simulink model "D53_LKAS_JLU_20200909_1612"  (R2018b)
settings: Solver=ode3  StartTime=0.0  StopTime=10.0  FixedStep=0.01  RelTol=1e-3  EnableMultiTasking=on
model workspace (MAT data in the model file):
  MCOS : class17 (value not decoded)
  MCOS : class17 (value not decoded)
  MCOS : class17 (value not decoded)
  MCOS : class17 (value not decoded)
  MCOS : class17 (value not decoded)
  MCOS : class17 (value not decoded)
  MCOS : class17 (value not decoded)
  MCOS : class17 (value not decoded)
  MCOS : class17 (value not decoded)
  MCOS : class17 (value not decoded)
  MCOS : class17 (value not decoded)
  MCOS : class17 (value not decoded)
  MCOS : class17 (value not decoded)
  MCOS : class17 (value not decoded)
  MCOS : class17 (value not decoded)
  MCOS : class17 (value not decoded)
  MCOS : class17 (value not decoded)
  MCOS : class17 (value not decoded)
  MCOS : class17 (value not decoded)
  MCOS : class17 (value not decoded)
  MCOS : class17 (value not decoded)
  MCOS : class17 (value not decoded)
  MCOS : class17 (value not decoded)
  MCOS : class17 (value not decoded)
  MCOS : class17 (value not decoded)
  MCOS : class17 (value not decoded)
  MCOS : class17 (value not decoded)
  MCOS : class17 (value not decoded)
  MCOS : class17 (value not decoded)
  MCOS : class17 (value not decoded)
  MCOS : class17 (value not decoded)
  MCOS : class17 (value not decoded)
  MCOS : class17 (value not decoded)
  MCOS : class17 (value not decoded)
  MCOS : class17 (value not decoded)
  MCOS : class17 (value not decoded)
  MCOS : class17 (value not decoded)
  MCOS : class17 (value not decoded)
  MCOS : class17 (value not decoded)
  MCOS : class17 (value not decoded)
  MCOS : class17 (value not decoded)
  MCOS : class17 (value not decoded)
  MCOS : class17 (value not decoded)
  MCOS : class17 (value not decoded)
  MCOS : class17 (value not decoded)
  MCOS : class17 (value not decoded)
  MCOS : class17 (value not decoded)
  MCOS : class17 (value not decoded)
  MCOS : class17 (value not decoded)
  MCOS : class17 (value not decoded)
  MCOS : class17 (value not decoded)
  MCOS : class17 (value not decoded)
  MCOS : class17 (value not decoded)
  MCOS : class17 (value not decoded)
  MCOS : class17 (value not decoded)
  MCOS : class17 (value not decoded)
  MCOS : class17 (value not decoded)
  MCOS : class17 (value not decoded)
  MCOS : class17 (value not decoded)
  MCOS : class17 (value not decoded)
  MCOS : class17 (value not decoded)
  MCOS : class17 (value not decoded)
  MCOS : class17 (value not decoded)
  MCOS : class17 (value not decoded)
  MCOS : class17 (value not decoded)
  MCOS : class17 (value not decoded)
  MCOS : class17 (value not decoded)
  MCOS : class17 (value not decoded)
  MCOS : class17 (value not decoded)
  MCOS : class17 (value not decoded)
  MCOS : class17 (value not decoded)
  MCOS : class17 (value not decoded)
  MCOS : class17 (value not decoded)
  MCOS : class17 (value not decoded)
  MCOS : class17 (value not decoded)
  MCOS : class17 (value not decoded)
  MCOS : class17 (value not decoded)
  MCOS : class17 (value not decoded)
  MCOS : class17 (value not decoded)
  MCOS : class17 (value not decoded)
  MCOS : class17 (value not decoded)
  MCOS : class17 (value not decoded)
  MCOS : class17 (value not decoded)
  MCOS : class17 (value not decoded)
  MCOS : class17 (value not decoded)
  MCOS : class17 (value not decoded)
  MCOS : class17 (value not decoded)
  MCOS : class17 (value not decoded)
  MCOS : class17 (value not decoded)
undefined symbols (not defined in the file): LKA_CarWidth, LKA_SampleTime, LKA_StrRatio_C, LKA_Veh2CamL_C, LKA_Veh2CamW_C, LKA_WhlBaseL_C, LL_CompSWA_C, LL_CrvtPrvwT_C, LL_DesDvt_C, LL_DvtComp_C, LL_DvtPrvwT_C, LL_DvtSpdDet_vDvtSpdMin_C, LL_HdAgExT_C, LL_HdAgPrvwT_C, LL_LAccMax_C, LL_LAccRMax_C, LL_LDW_EarliestWarnLine_C, LL_LDW_LatestWarnLine_C, LL_LDWS_SUPPRESS_HEADING, LL_LFClb_TFC_DiffCtlBalance, LL_LFClb_TFC_DiffCtrlMaxSWA, LL_LFClb_TFC_DiffCtrlRatio, LL_LFClb_TFC_facmGainLutGain1_C, LL_LFClb_TFC_facmGainLutGain2_C, LL_LFClb_TFC_facmIntegRatio, LL_LFClb_TFC_facmKlat_C, LL_LFClb_TFC_FfCtlRatio_C, LL_LFClb_TFC_phiIntegCtlMaxSWA_C, LL_LFClb_TFC_tiKlatPrvwT_C, LL_LFClb_TFC_vGainLutVehSpdLwr_C, LL_LFClb_TFC_vGainLutVehSpdUpr_C, LL_LKA_EarliestWarnLine_C, LL_LKA_LatestWarnLine_C, LL_LKAExPrcs_ExitC0Dvt, LL_LKAExPrcs_ExitC0Swt, LL_LKAExPrcs_tiExitTime1, LL_LKAExPrcs_tiExitTime2, LL_LKAExPrcs_tiExitTime3, LL_LKAS_OUT_OF_CONTROL_LAT_VEL, LL_LKAS_OUT_OF_CONTROL_TTLC, LL_LKASWASyn_M0, LL_LKASWASyn_M1, LL_LKASWASyn_M2, LL_LKASWASyn_M3K, LL_LKASWASyn_SWAaddMax, LL_LKASWASyn_T2, LL_LKASWASyn_tiTrqSwaRtTime, LL_LKASWASyn_tiTrqSwaTime, LL_LKASWASyn_TrqMax, LL_LKASWASyn_TrqSwaAddSwt, LL_LKASWASyn_TrqSwaRateDiff, LL_LSpdCompT_C, LL_lStpLngth_C, LL_MAX_DELAY_EPSSTAR_TIME, LL_MAX_DRIVER_TORQUE_DISABLE, LL_MAX_DRIVER_TORQUE_ENABLE, LL_MAX_LANE_WIDTH_DISABLE, LL_MAX_LANE_WIDTH_ENABLE, LL_MAX_LAT_ACC_DISABLE, LL_MAX_LAT_ACC_ENABLE ... (+30)
libraries: simulink x134, canmsglib x50, dspstat3 x3, simulink_extras x1
(part 7 of 17)

== system D53_LKAS_JLU_20200909_1612/LL/LL Inputs Mapping/bsVehMovInfo ==
  bsVehMovInfoIn : Inport
  Bus Creator : BusCreator  Inputs=10
  Bus Selector2 : BusSelector  OutputSignals=ESC_LatAcc,ESC_LatAcc_Valid,ESC_YawRate,ESC_YawRate_Valid,ESC_UnYawRate,ESC_VehSpd,ESC_LonAcc,ESC_LonAcc_Valid,ESC_Brake_Press,ESC_VehSpd_Valid
  bsVehMovInfoOut : Outport
  wires:
  bsVehMovInfoIn/1 -> Bus Selector2/1
  Bus Selector2/1 -> Bus Creator/1  "<ESC_LatAcc>"
  Bus Selector2/2 -> Bus Creator/2  "<ESC_LatAcc_Valid>"
  Bus Selector2/3 -> Bus Creator/3  "<ESC_YawRate>"
  Bus Selector2/4 -> Bus Creator/4  "<ESC_YawRate_Valid>"
  Bus Selector2/5 -> Bus Creator/5  "<ESC_UnYawRate>"
  Bus Selector2/6 -> Bus Creator/6  "<ESC_VehSpd>"
  Bus Selector2/7 -> Bus Creator/7  "<ESC_LonAcc>"
  Bus Selector2/8 -> Bus Creator/8  "<ESC_LonAcc_Valid>"
  Bus Selector2/9 -> Bus Creator/9  "<ESC_Brake_Press>"
  Bus Selector2/10 -> Bus Creator/10  "<ESC_VehSpd_Valid>"
  Bus Creator/1 -> bsVehMovInfoOut/1

== system D53_LKAS_JLU_20200909_1612/LL/LLOn/LDW ==
  LDW_stLDWActvFlg : Inport
  LDW_bsInInfoSyn : Inport  Port=2
  LDW_bsLDWClb : Inport  Port=3
  states : EnablePort  StatesWhenEnabling=reset
      settings: AttributesFormatString=states = %<StatesWhenEnabling>
  Bus Selector : BusSelector  OutputSignals=bsLaneInfo.bsL0Info.L0_C1,bsLaneInfo.bsR0Info.R0_C1
  Bus Selector1 : BusSelector  OutputSignals=LL_LDWS_SUPPRESS_HEADING
  Heading Angle Detection (HdAgDet) : Subsystem  Description=|
      | Block Name: Heading Angle Detection
      | Ab.: HdAgDet
      | No.: 1.3.1.0
      | Rev: 0.0.1
      | Update Date: 19-3-26
  LDWWarnInfo : MATLAB Function  TreatAsAtomicUnit=on
  LDW_Flag : Outport  OutputWhenDisabled=reset  InitialOutput=0
  wires:
  LDWWarnInfo/1(LDWWarnInfo) -> LDW_Flag/1
  Heading Angle Detection (HdAgDet)/1(HdAgDet_stHdAgDetFlg) -> LDWWarnInfo/2(LDW_stHdAgDetFlg)
  Bus Selector1/1 -> Heading Angle Detection (HdAgDet)/4(HdAgDet_phiHdAgThres_C)  "<LL_LDWS_SUPPRESS_HEADING>"
  LDW_bsLDWClb/1 -> Bus Selector1/1
  Bus Selector/2 -> Heading Angle Detection (HdAgDet)/3(HdAgDet_phiHdAgRgt)  "<R0_C1>"
  Bus Selector/1 -> Heading Angle Detection (HdAgDet)/2(HdAgDet_phiHdAgLft)  "<L0_C1>"
  LDW_stLDWActvFlg/1 -> LDWWarnInfo/1(LDW_stLDWActvFlg), Heading Angle Detection (HdAgDet)/1(HdAgDet_stLDWActvFlg)
  LDW_bsInInfoSyn/1 -> Bus Selector/1

== system D53_LKAS_JLU_20200909_1612/LL/LLOn/LKA ==
  LKA_bsInInfoSyn : Inport
  LKA_bsLKAInPInfo : Inport  Port=2
  LKA_bsLKAClb : Inport  Port=3
  LKA_bsConstantClb : Inport  Port=4
  states = reset : EnablePort  StatesWhenEnabling=reset  ShowOutputPort=on
  Bus Selector : BusSelector  OutputSignals=LKA_SampleTime
  Cast To Single : DataTypeConversion  OutDataTypeStr=uint8
  Driver Torque Addition (DTA) : Subsystem
  LKA Exit Processing (LKAExPrcs) : Subsystem  Description=|
      | Block Name: LKA Exit Processing 
      | Ab.: LKAExPrcs
      | No.: 1.2.2.0
      | Rev: 0.0.1
      | Update Date: 19-5-13
  "LKA Motion Planning (LKAMP) " : Subsystem  Description=|
      | Block Name: LKA Motion Planning
      | Ab.: LKAMP
      | No.: 1.2.3.0
      | Rev: 0.0.1
      | Update Date: 19-5-13
  LKA SWA Limit (LKASWALim) : Subsystem  Description=|
      | Block Name: LKA SWA Synthesis
      | Ab.: LKASWASyn
      | No.: 1.2.6.0
      | Rev: 0.0.1
      | Update Date: 19-5-13
  LKA_Mon : Subsystem
  Lane Following (LF) : Subsystem  Description=|
      | Block Name: Lane Following
      | Ab.: LF
      | No.: 02
      | Rev: 00.00.01
      | Update Date: 19-3-28
  Plan To LaneFollowing (PTLF) : Subsystem
  LKA_ExitFlg : Outport  OutputWhenDisabled=reset  InitialOutput=0
  LKA_phiSWACmd : Outport  Port=2  OutputWhenDisabled=reset  InitialOutput=0
  LKA_M : Outport  Port=3  OutputWhenDisabled=reset  InitialOutput=0
  LKAMon : Outport  Port=4  OutputWhenDisabled=reset  InitialOutput=0
  tag scope: ActFlg=global, Ff=global, LKA_ConstantClb=global, LKA_ExitFlg_Mon=global, LKA_SampleTime=global, PT1=global
  wires:
  LKA_Mon/1(LKAMon) -> LKAMon/1
  "LKA Motion Planning (LKAMP) "/2(LKAMP_tiT1) -> [PT1]  "PlanT1"
  "LKA Motion Planning (LKAMP) "/3(LKAMP_tiT2) -> ?  "PlanT2"
  "LKA Motion Planning (LKAMP) "/1(LKAMP_phiSWACmd) -> [Plan]  "PlanSWACmd"
  Lane Following (LF)/4(LF_phiDiffSWACmd) -> [D]
  Lane Following (LF)/2(LF_phiPropSWACmd) -> [P]
  Lane Following (LF)/1(LF_phiFfLFSWACmd) -> [Ff]
  Lane Following (LF)/3(LF_phiIntegSWACmd) -> [I]
  Driver Torque Addition (DTA)/2(DTA_M) -> LKA_M/1
  [LKAInPInfo] -> Lane Following (LF)/2(LF_bsLKAInPInfo)
  [Ff] -> LKA SWA Limit (LKASWALim)/2(LKASWALim_Ff)
  [LKA_bsInInfoSyn] -> Lane Following (LF)/1(LF_bsInInfoSyn)
  [LKA_bsInInfoSyn] -> Driver Torque Addition (DTA)/1(DTA_bsInInfoSyn)
  [LKA_bsInInfoSyn] -> "LKA Motion Planning (LKAMP) "/1(LKAMP_bsInInfoSyn)
  [LKA_bsInInfoSyn] -> LKA Exit Processing (LKAExPrcs)/1(LKAExPrcs_bsInInfoSyn)
  LKA_bsInInfoSyn/1 -> [LKA_bsInInfoSyn]
  [LKA_bsLKAClb] -> LKA SWA Limit (LKASWALim)/4(LKASWALim_bsLKAClb)
  [LKA_bsLKAClb] -> Lane Following (LF)/3(LF_bsLFClb)
  [LKA_bsLKAClb] -> Driver Torque Addition (DTA)/2(DTA_bsLFClb)
  [LKA_bsLKAClb] -> "LKA Motion Planning (LKAMP) "/4(LKAMP_bsLKAClb)
  [LKA_bsLKAClb] -> LKA Exit Processing (LKAExPrcs)/3(LKAExPrcs_bsLKAClb)
  [LKAInPInfo] -> LKA SWA Limit (LKASWALim)/3(LKASWALim_bsLKAInPInfo)
  LKA_bsLKAClb/1 -> [LKA_bsLKAClb]
  [LKAInPInfo] -> Plan To LaneFollowing (PTLF)/1(InP)
  [LKAInPInfo] -> LKA Exit Processing (LKAExPrcs)/2(LKAExPrcs_bsLKAInPInfo)
  [LKAInPInfo] -> "LKA Motion Planning (LKAMP) "/3(LKAMP_bsLKAInPInfo)
  LKA_bsLKAInPInfo/1 -> [LKAInPInfo]
  [LKA_ConstantClb] -> Lane Following (LF)/4(LF_bsConstantClb)
  [LKA_ConstantClb] -> "LKA Motion Planning (LKAMP) "/5(LLClb_bsConstantClb)
  [ActFlg] -> "LKA Motion Planning (LKAMP) "/2(LKAMP_stLKAActvFlg)
  [PT1] -> LKA Exit Processing (LKAExPrcs)/4(LKAExPrcs_PlanT1)
  [PT1] -> Plan To LaneFollowing (PTLF)/3(T1)
  [Plan] -> Plan To LaneFollowing (PTLF)/2(Plan)
  [DT] -> Plan To LaneFollowing (PTLF)/4(DrvTrq)
  Driver Torque Addition (DTA)/1(DTA_phiDTASWACmd) -> [DT]  "DT"
  [D] -> Plan To LaneFollowing (PTLF)/8(D)
  [I] -> Plan To LaneFollowing (PTLF)/7(I)
  [P] -> Plan To LaneFollowing (PTLF)/6(P)
  [Ff] -> Plan To LaneFollowing (PTLF)/5(Ff)
  LKA Exit Processing (LKAExPrcs)/1(LKAExPrcs_stExFlg) -> LKA_ExitFlg/1, [LKA_ExitFlg_Mon]
  LKA SWA Limit (LKASWALim)/1(LKASWALim_phiSWACmd) -> LKA_phiSWACmd/1  "phiSWACmd"
  states = reset/1 -> Cast To Single/1
  Plan To LaneFollowing (PTLF)/1(SWACmd) -> LKA SWA Limit (LKASWALim)/1(LKASWALim_phiTFCSWACmd)  "PTLFSWACmd"
  Cast To Single/1 -> [ActFlg]  "ActFlg"
  LKA_bsConstantClb/1 -> [LKA_ConstantClb], Bus Selector/1
  Bus Selector/1 -> [LKA_SampleTime]  "<LKA_SampleTime>"

== system D53_LKAS_JLU_20200909_1612/LL/LLOn/LKA Input Processing (LKAInP) ==
  LKAInP_stLKAActvFlg : Inport
  LKAInP_bsInInfoSyn : Inport  Port=2
  LKAInP_bsLKAClb : Inport  Port=3
  Bus Creator : BusCreator  Inputs=6
  Bus Creator1 : BusCreator  Inputs=3
  Delay : Delay  DelayLength=1
  Lane Width Calculation (LW) : Subsystem
  Predicted Deviation Calculation (PrDvt) : Subsystem
  Predicted Heading Angle Calculation (PrHdAg) : Subsystem
  Previewed Curvature (PrCrvt) : Subsystem
  Steering Wheel Position Calculation (SWAPosCal) : Subsystem
  TTLC Calculation (TTLCCalc) : Subsystem  Description=|
      | Block Name: TTLC Calculation
      | Ab.: TTLCCalc
      | No.: 1.1.1.1
      | Rev: 0.0.1
      | Update Date: 19-3-26
  Under The Limit (UndrLim) : Subsystem
  LKAInP_bsLKAInPInfo : Outport
  wires:
  TTLC Calculation (TTLCCalc)/1(TTLCCalc_bsTTLCInfo) -> Predicted Heading Angle Calculation (PrHdAg)/1(PrHdAg_bsTTLCInfo), Bus Creator/2  "TTLC_bsTTLCInfo"
  Lane Width Calculation (LW)/1(LW_LaneWidth) -> Bus Creator/1  "LW_LaneWidth"
  Steering Wheel Position Calculation (SWAPosCal)/1(SWAPosCal) -> Bus Creator/6  "LKAInP_phiSWAPos"
  LKAInP_stLKAActvFlg/1 -> Delay/1
  Under The Limit (UndrLim)/2(UndrLim_dphiSWARMax) -> Bus Creator/5  "UndrLim_dphiSWARMax"
  Under The Limit (UndrLim)/1(UndrLim_phiSWAMax) -> Bus Creator/4  "UndrLim_phiSWAMax"
  Bus Creator1/1 -> Bus Creator/3  "Pr_bsPrInfo"
  Previewed Curvature (PrCrvt)/1(PrvwCrvt_bsPrvwCrvtInfo) -> Bus Creator1/3, TTLC Calculation (TTLCCalc)/3(bsPrvwCrvtInfo)  "bsPrCrvtInfo"
  Predicted Deviation Calculation (PrDvt)/1(PrdcDvt_bsPrdcDvtInfo) -> Bus Creator1/1, TTLC Calculation (TTLCCalc)/2(bsPrDvtInfo)  "bsPrDvtInfo"
  Predicted Heading Angle Calculation (PrHdAg)/1(PrHdAg_bsPrHdAgInfo) -> Bus Creator1/2, Predicted Deviation Calculation (PrDvt)/3(PrdcDvt_bsPrdcHdAgInfo)  "bsPrHdAgInfo"
  LKAInP_bsLKAClb/1 -> Predicted Deviation Calculation (PrDvt)/4(PrdcDvt_bsLKAClb), Predicted Heading Angle Calculation (PrHdAg)/4(PrHdAg_bsLKAClb), Previewed Curvature (PrCrvt)/3(PrvwCrvt_tiCrvtPrvwT_C), Under The Limit (UndrLim)/2(UndrLim_bsUndrLimClb)
  Bus Creator/1 -> LKAInP_bsLKAInPInfo/1
  LKAInP_bsInInfoSyn/1 -> Lane Width Calculation (LW)/1(LW_bsInInfoSyn), TTLC Calculation (TTLCCalc)/1(bsInfo), Predicted Deviation Calculation (PrDvt)/2(PrdcDvt_bsInInfoSyn), Predicted Heading Angle Calculation (PrHdAg)/3(PrHdAg_bsInInfoSyn), Previewed Curvature (PrCrvt)/2(PrvwCrvt_bsInInfoSyn), Under The Limit (UndrLim)/1(UndrLim_bsInInfoSyn), Steering Wheel Position Calculation (SWAPosCal)/1(SWAPosCal_bsInInfoSyn)
  Delay/1 -> Predicted Deviation Calculation (PrDvt)/1(PrdcDvt_stLKAActvFlg), Predicted Heading Angle Calculation (PrHdAg)/2(PrdcHdAg_stLKAActvFlg), Previewed Curvature (PrCrvt)/1(PrvwCrvt_stLKAActvFlg)

== system D53_LKAS_JLU_20200909_1612/LL/LLOn/LL State Determination (LLStateDet) ==
  LLStateDet_stDACMode : Inport
  LLStateDet_bsInInfoSyn : Inport  Port=2
  LLStateDet_bsLKAInPInfo : Inport  Port=3
  LLStateDet_bsLLSMConClb : Inport  Port=4
  LLStateDet_stExitFlg : Inport  Port=5
  LLStateDet_SignalFault : Inport  Port=6
  Bus Creator : BusCreator  Inputs=3
  Delay : Delay  DelayLength=1
  Delay1 : Delay  DelayLength=1
  LDW_State_Machine : Stateflow chart  Description=|  TreatAsAtomicUnit=on
      | Block Name: LDW State Machine
      | Ab.: LDWSM
      | No.: 1.1.2.0
      | Rev: 0.0.1
      | Update Date: 19-3-26
      settings: RTWSystemCode=Nonreusable function
  LKA_State_Machine : Stateflow chart  Description=|  TreatAsAtomicUnit=on
      | Block Name: LKA State Machine
      | Ab.: LKASM
      | No.: 1.1.3.0
      | Rev: 0.0.1
      | Update Date: 19-3-26
      settings: RTWSystemCode=Nonreusable function
  LL State Machine Conditions (LLSMCon) : Subsystem
  LLStateDet_bsLLState : Outport
  LLStateDet_stLDWActvFlg : Outport  Port=2
  LLStateDet_stLKAActvFlg : Outport  Port=3
  tag scope: LDW_State_Mon=global, LKA_State_Mon=global
  wires:
  LLStateDet_SignalFault/1 -> LL State Machine Conditions (LLSMCon)/7(LLSMCon_bsSignalFault)
  Delay/1 -> LL State Machine Conditions (LLSMCon)/6(LLSMCon_stExitFlg)
  LLStateDet_bsLLSMConClb/1 -> LL State Machine Conditions (LLSMCon)/4(LLSMCon_bsLLSMConClb)
  LLStateDet_stExitFlg/1 -> Delay/1
  LLStateDet_stDACMode/1 -> LL State Machine Conditions (LLSMCon)/1(LLSMCon_stDACModeIn)
  LLStateDet_bsLKAInPInfo/1 -> LL State Machine Conditions (LLSMCon)/3(LLSMCon_bsLKAInPInfo)
  LLStateDet_bsInInfoSyn/1 -> LL State Machine Conditions (LLSMCon)/2(LLSMCon_bsInInfoSyn)
  LL State Machine Conditions (LLSMCon)/11(LLSMCon_stLKAFaultCSyn) -> LKA_State_Machine/6(LKASM_stFaultCSyn)
  LL State Machine Conditions (LLSMCon)/10(LLSMCon_stLKADeactvCSyn) -> LKA_State_Machine/5(LKASM_stDeactvCSyn)
  LL State Machine Conditions (LLSMCon)/9(LLSMCon_stLKAActvCSyn) -> LKA_State_Machine/4(LKASM_stActvCSyn)
  LL State Machine Conditions (LLSMCon)/8(LLSMCon_stLKADisblCSyn) -> LKA_State_Machine/3(LKASM_stDisblCSyn)
  LL State Machine Conditions (LLSMCon)/7(LLSMCon_stLKAEnaCSyn) -> LKA_State_Machine/2(LKASM_stEnaCSyn)
  LL State Machine Conditions (LLSMCon)/6(LLSMCon_stLDWFaultCSyn) -> LDW_State_Machine/6(LDWSM_stFaultCSyn)
  LDW_State_Machine/2(LDWSM_stLDWState) -> Bus Creator/1, [LDW_State_Mon]  "LDW_State"
  LKA_State_Machine/2(LKASM_stLKAState) -> Bus Creator/3, [LKA_State_Mon]  "LKA_State"
  Bus Creator/1 -> LLStateDet_bsLLState/1, Delay1/1  "LLState"
  Delay1/1 -> LL State Machine Conditions (LLSMCon)/5(LLSMCon_bsLLState)
  LKA_State_Machine/1(LKASM_stLKAActvFlg) -> LLStateDet_stLKAActvFlg/1
  LDW_State_Machine/1(LDWSM_stLDWActvFlg) -> LLStateDet_stLDWActvFlg/1
  LL State Machine Conditions (LLSMCon)/1(LLSMCon_stDACMode) -> LDW_State_Machine/1(LDWSM_stLMCMode), Bus Creator/2, LKA_State_Machine/1(LKASM_stLMCMode)  "DACMode"
  LL State Machine Conditions (LLSMCon)/5(LLSMCon_stLDWDeactvCSyn) -> LDW_State_Machine/5(LDWSM_stDeactvCSyn)
  LL State Machine Conditions (LLSMCon)/4(LLSMCon_stLDWActvCSyn) -> LDW_State_Machine/4(LDWSM_stActvCSyn)
  LL State Machine Conditions (LLSMCon)/3(LLSMCon_stLDWDisblCSyn) -> LDW_State_Machine/3(LDWSM_stDisblCSyn)
  LL State Machine Conditions (LLSMCon)/2(LLSMCon_stLDWEnaCSyn) -> LDW_State_Machine/2(LDWSM_stEnaCSyn)

== system D53_LKAS_JLU_20200909_1612/LL/LLOn/LL_Mon ==
  LKAMon : Inport
  Bus : BusCreator  Inputs=3
  BusInP : BusCreator  Inputs=2
  BusState : BusCreator  Inputs=2
  LLMon : Outport
  wires:
  BusState/1 -> [StateMon]  "StateMon"
  BusInP/1 -> [InPMon]  "InPMon"
  [LKA_State_Mon] -> BusState/2  "LKA_State_Mon"
  [LDW_State_Mon] -> BusState/1  "LDW_State_Mon"
  [RGTTTLC_Mon] -> BusInP/2  "RGTTTLC_Mon"
  [LFTTTLC_Mon] -> BusInP/1  "LFTTTLC_Mon"
  Bus/1 -> LLMon/1  "LLMon"
  LKAMon/1 -> Bus/3
  [StateMon] -> Bus/2
  [InPMon] -> Bus/1

== system D53_LKAS_JLU_20200909_1612/LLClb/LLSMConClb/ICv to v ==
  In1 : Inport
  Add : Sum  Inputs=+-
  Constant : Constant  Value=2.5  OutDataTypeStr=single
  Gain : Gain  Gain=1/1.02
  Out1 : Outport
  wires:
  Gain/1 -> Out1/1
  Constant/1 -> Add/2
  Add/1 -> Gain/1
  In1/1 -> Add/1

== system D53_LKAS_JLU_20200909_1612/LLClb/LLSMConClb/ICv to v1 ==
  In1 : Inport
  Add : Sum  Inputs=+-
  Constant : Constant  Value=2.5  OutDataTypeStr=single
  Gain : Gain  Gain=1/1.02
  Out1 : Outport
  wires:
  In1/1 -> Add/1
  Add/1 -> Gain/1
  Constant/1 -> Add/2
  Gain/1 -> Out1/1

== system D53_LKAS_JLU_20200909_1612/LLClb/LLSMConClb/ICv to v2 ==
  In1 : Inport
  Add : Sum  Inputs=+-
  Constant : Constant  Value=2.5  OutDataTypeStr=single
  Gain : Gain  Gain=1/1.02
  Out1 : Outport
  wires:
  Gain/1 -> Out1/1
  Constant/1 -> Add/2
  Add/1 -> Gain/1
  In1/1 -> Add/1

== system D53_LKAS_JLU_20200909_1612/LLClb/LLSMConClb/ICv to v3 ==
  In1 : Inport
  Add : Sum  Inputs=+-
  Constant : Constant  Value=2.5  OutDataTypeStr=single
  Gain : Gain  Gain=1/1.02
  Out1 : Outport
  wires:
  In1/1 -> Add/1
  Add/1 -> Gain/1
  Constant/1 -> Add/2
  Gain/1 -> Out1/1

== system D53_LKAS_JLU_20200909_1612/LLClb/LLSMConClb/ICv to v4 ==
  In1 : Inport
  Add : Sum  Inputs=+-
  Constant : Constant  Value=2.5  OutDataTypeStr=single
  Gain : Gain  Gain=1/1.02
  Out1 : Outport
  wires:
  Gain/1 -> Out1/1
  Constant/1 -> Add/2
  Add/1 -> Gain/1
  In1/1 -> Add/1

== system D53_LKAS_JLU_20200909_1612/LLClb/LLSMConClb/ICv to v5 ==
  In1 : Inport
  Add : Sum  Inputs=+-
  Constant : Constant  Value=2.5  OutDataTypeStr=single
  Gain : Gain  Gain=1/1.02
  Out1 : Outport
  wires:
  In1/1 -> Add/1
  Add/1 -> Gain/1
  Constant/1 -> Add/2
  Gain/1 -> Out1/1

== system D53_LKAS_JLU_20200909_1612/Clb/Calibration1/Subsystem2/If Action Subsystem ==
  In1 : Inport
  Action Port : ActionPort  ActionType=then
  Out1 : Outport
  wires:
  In1/1 -> Out1/1

== system D53_LKAS_JLU_20200909_1612/Clb/Calibration1/Subsystem2/If Action Subsystem1 ==
  In1 : Inport
  Action Port : ActionPort  ActionType=elseif
  Out1 : Outport
  wires:
  In1/1 -> Out1/1

== system D53_LKAS_JLU_20200909_1612/Clb/Calibration1/Subsystem2/If Action Subsystem2 ==
  In1 : Inport
  Action Port : ActionPort  ActionType=elseif
  Out1 : Outport
  wires:
  In1/1 -> Out1/1

== system D53_LKAS_JLU_20200909_1612/Clb/Calibration1/Subsystem2/If Action Subsystem3 ==
  In1 : Inport
  Action Port : ActionPort  ActionType=elseif
  Out1 : Outport
  wires:
  In1/1 -> Out1/1

== system D53_LKAS_JLU_20200909_1612/Clb/Calibration1/Subsystem2/If Action Subsystem4 ==
  In1 : Inport
  Action Port : ActionPort  ActionType=elseif
  Out1 : Outport
  wires:
  In1/1 -> Out1/1

== system D53_LKAS_JLU_20200909_1612/Clb/Calibration1/Subsystem2/If Action Subsystem5 ==
  In1 : Inport
  Action Port : ActionPort  ActionType=elseif
  Out1 : Outport
  wires:
  In1/1 -> Out1/1

== system D53_LKAS_JLU_20200909_1612/Clb/Calibration1/Subsystem2/If Action Subsystem6 ==
  In1 : Inport
  Action Port : ActionPort  ActionType=elseif
  Out1 : Outport
  wires:
  In1/1 -> Out1/1

== system D53_LKAS_JLU_20200909_1612/Clb/Calibration1/Subsystem2/If Action Subsystem7 ==
  In1 : Inport
  Action Port : ActionPort  ActionType=elseif
  Out1 : Outport
  wires:
  In1/1 -> Out1/1

== system D53_LKAS_JLU_20200909_1612/Clb/Calibration1/Subsystem2/If Action Subsystem8 ==
  In1 : Inport
  Action Port : ActionPort  ActionType=elseif
  Out1 : Outport
  wires:
  In1/1 -> Out1/1

== system D53_LKAS_JLU_20200909_1612/Clb/Calibration1/Subsystem2/If Action Subsystem9 ==
  In1 : Inport
  Action Port : ActionPort  ActionType=elseif
  Out1 : Outport
  wires:
  In1/1 -> Out1/1

== system D53_LKAS_JLU_20200909_1612/Clb/Calibration2/Subsystem2/If Action Subsystem ==
  In1 : Inport
  Action Port : ActionPort  ActionType=then
  Out1 : Outport
  wires:
  In1/1 -> Out1/1

== system D53_LKAS_JLU_20200909_1612/Clb/Calibration2/Subsystem2/If Action Subsystem1 ==
  In1 : Inport
  Action Port : ActionPort  ActionType=elseif
  Out1 : Outport
  wires:
  In1/1 -> Out1/1

== system D53_LKAS_JLU_20200909_1612/Clb/Calibration2/Subsystem2/If Action Subsystem2 ==
  In1 : Inport
  Action Port : ActionPort  ActionType=elseif
  Out1 : Outport
  wires:
  In1/1 -> Out1/1

== system D53_LKAS_JLU_20200909_1612/Clb/Calibration2/Subsystem2/If Action Subsystem3 ==
  In1 : Inport
  Action Port : ActionPort  ActionType=elseif
  Out1 : Outport
  wires:
  In1/1 -> Out1/1

== system D53_LKAS_JLU_20200909_1612/Clb/Calibration2/Subsystem2/If Action Subsystem4 ==
  In1 : Inport
  Action Port : ActionPort  ActionType=elseif
  Out1 : Outport
  wires:
  In1/1 -> Out1/1

== system D53_LKAS_JLU_20200909_1612/Clb/Calibration2/Subsystem2/If Action Subsystem5 ==
  In1 : Inport
  Action Port : ActionPort  ActionType=elseif
  Out1 : Outport
  wires:
  In1/1 -> Out1/1

== system D53_LKAS_JLU_20200909_1612/Clb/Calibration2/Subsystem2/If Action Subsystem6 ==
  In1 : Inport
  Action Port : ActionPort  ActionType=elseif
  Out1 : Outport
  wires:
  In1/1 -> Out1/1

== system D53_LKAS_JLU_20200909_1612/Clb/Calibration2/Subsystem2/If Action Subsystem7 ==
  In1 : Inport
  Action Port : ActionPort  ActionType=elseif
  Out1 : Outport
  wires:
  In1/1 -> Out1/1

== system D53_LKAS_JLU_20200909_1612/Clb/Calibration2/Subsystem2/If Action Subsystem8 ==
  In1 : Inport
  Action Port : ActionPort  ActionType=elseif
  Out1 : Outport
  wires:
  In1/1 -> Out1/1

== system D53_LKAS_JLU_20200909_1612/Clb/Calibration2/Subsystem2/If Action Subsystem9 ==
  In1 : Inport
  Action Port : ActionPort  ActionType=elseif
  Out1 : Outport
  wires:
  In1/1 -> Out1/1

== system D53_LKAS_JLU_20200909_1612/Clb/Calibration3/Subsystem2/If Action Subsystem ==
  In1 : Inport
  Action Port : ActionPort  ActionType=then
  Out1 : Outport
  wires:
  In1/1 -> Out1/1

== system D53_LKAS_JLU_20200909_1612/Clb/Calibration3/Subsystem2/If Action Subsystem1 ==
  In1 : Inport
  Action Port : ActionPort  ActionType=elseif
  Out1 : Outport
  wires:
  In1/1 -> Out1/1

== system D53_LKAS_JLU_20200909_1612/Clb/Calibration3/Subsystem2/If Action Subsystem2 ==
  In1 : Inport
  Action Port : ActionPort  ActionType=elseif
  Out1 : Outport
  wires:
  In1/1 -> Out1/1

== system D53_LKAS_JLU_20200909_1612/Clb/Calibration3/Subsystem2/If Action Subsystem3 ==
  In1 : Inport
  Action Port : ActionPort  ActionType=elseif
  Out1 : Outport
  wires:
  In1/1 -> Out1/1

== system D53_LKAS_JLU_20200909_1612/Clb/Calibration3/Subsystem2/If Action Subsystem4 ==
  In1 : Inport
  Action Port : ActionPort  ActionType=elseif
  Out1 : Outport
  wires:
  In1/1 -> Out1/1

== system D53_LKAS_JLU_20200909_1612/Clb/Calibration3/Subsystem2/If Action Subsystem5 ==
  In1 : Inport
  Action Port : ActionPort  ActionType=elseif
  Out1 : Outport
  wires:
  In1/1 -> Out1/1

== system D53_LKAS_JLU_20200909_1612/Clb/Calibration3/Subsystem2/If Action Subsystem6 ==
  In1 : Inport
  Action Port : ActionPort  ActionType=elseif
  Out1 : Outport
  wires:
  In1/1 -> Out1/1

== system D53_LKAS_JLU_20200909_1612/Clb/Calibration3/Subsystem2/If Action Subsystem7 ==
  In1 : Inport
  Action Port : ActionPort  ActionType=elseif
  Out1 : Outport
  wires:
  In1/1 -> Out1/1

== system D53_LKAS_JLU_20200909_1612/Clb/Calibration3/Subsystem2/If Action Subsystem8 ==
  In1 : Inport
  Action Port : ActionPort  ActionType=elseif
  Out1 : Outport
  wires:
  In1/1 -> Out1/1

== system D53_LKAS_JLU_20200909_1612/Clb/Calibration3/Subsystem2/If Action Subsystem9 ==
  In1 : Inport
  Action Port : ActionPort  ActionType=elseif
  Out1 : Outport
  wires:
  In1/1 -> Out1/1

== system D53_LKAS_JLU_20200909_1612/LL/Human Machine Interface (HMI)/Subsystem/Count 10s ==
  Enable : EnablePort  StatesWhenEnabling=reset
  Add : Sum
  Compare To Constant27 : simulink/Logic and Bit Operations/Compare To Constant  relop=>=  const=1000  OutDataTypeStr=boolean
  Constant : Constant  OutDataTypeStr=uint16
  Memory : Memory  InheritSampleTime=on
  Saturation : Saturate  UpperLimit=2100  LowerLimit=0
  Out : Outport  OutputWhenDisabled=reset  InitialOutput=0
  wires:
  Compare To Constant27/1 -> Out/1
  Constant/1 -> Add/1
  Add/1 -> Saturation/1
  Saturation/1 -> Compare To Constant27/1, Memory/1
  Memory/1 -> Add/2

== system D53_LKAS_JLU_20200909_1612/LL/Human Machine Interface (HMI)/Subsystem/Count 15s ==
  Enable : EnablePort  StatesWhenEnabling=reset
  Add : Sum
  Compare To Constant27 : simulink/Logic and Bit Operations/Compare To Constant  relop=>=  const=1500  OutDataTypeStr=boolean
  Constant : Constant  OutDataTypeStr=uint16
  Memory : Memory  InheritSampleTime=on
  Saturation : Saturate  UpperLimit=2100  LowerLimit=0
  Out : Outport  OutputWhenDisabled=reset  InitialOutput=0
  wires:
  Memory/1 -> Add/2
  Saturation/1 -> Memory/1, Compare To Constant27/1
  Add/1 -> Saturation/1
  Constant/1 -> Add/1
  Compare To Constant27/1 -> Out/1

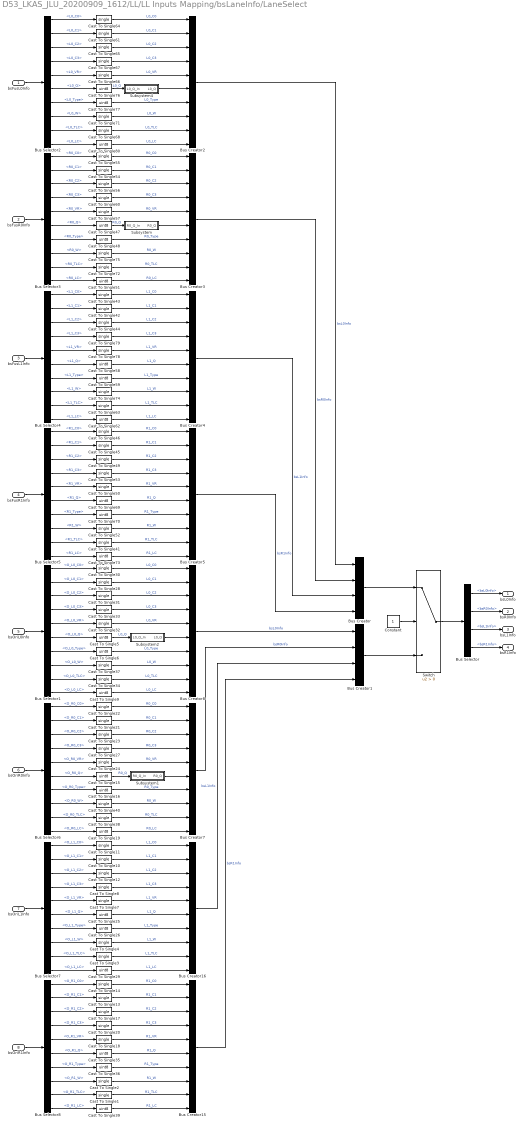
== system D53_LKAS_JLU_20200909_1612/LL/LL Inputs Mapping/bsLaneInfo/LaneSelect ==
  bsFusL0Info : Inport
  bsFusR0Info : Inport  Port=2
  bsFusL1Info : Inport  Port=3
  bsFusR1Info : Inport  Port=4
  bsOriL0Info : Inport  Port=5
  bsOriR0Info : Inport  Port=6
  bsOriL1Info : Inport  Port=7
  bsOriR1Info : Inport  Port=8
  Bus Creator : BusCreator  Inputs=4
  Bus Creator1 : BusCreator  Inputs=4
  Bus Creator{2..5,7..8,15..16} (8 alike) : BusCreator  Inputs=10
  Bus Selector : BusSelector  OutputSignals=bsL0Info,bsR0Info,bsL1Info,bsR1Info
  Bus Selector1 : BusSelector  OutputSignals=O_L0_C0,O_L0_C1,O_L0_C2,O_L0_C3,O_L0_VR,O_L0_Q,O_L0_Type,O_L0_W,O_L0_TLC,O_L0_LC
  Bus Selector2 : BusSelector  OutputSignals=L0_C0,L0_C1,L0_C2,L0_C3,L0_VR,L0_Q,L0_Type,L0_W,L0_TLC,L0_LC
  Bus Selector3 : BusSelector  OutputSignals=R0_C0,R0_C1,R0_C2,R0_C3,R0_VR,R0_Q,R0_Type,R0_W,R0_TLC,R0_LC
  Bus Selector4 : BusSelector  OutputSignals=L1_C0,L1_C1,L1_C2,L1_C3,L1_VR,L1_Q,L1_Type,L1_W,L1_TLC,L1_LC
  Bus Selector5 : BusSelector  OutputSignals=R1_C0,R1_C1,R1_C2,R1_C3,R1_VR,R1_Q,R1_Type,R1_W,R1_TLC,R1_LC
  Bus Selector6 : BusSelector  OutputSignals=O_R0_C0,O_R0_C1,O_R0_C2,O_R0_C3,O_R0_VR,O_R0_Q,O_R0_Type,O_R0_W,O_R0_TLC,O_R0_LC
  Bus Selector7 : BusSelector  OutputSignals=O_L1_C0,O_L1_C1,O_L1_C2,O_L1_C3,O_L1_VR,O_L1_Q,O_L1_Type,O_L1_W,O_L1_TLC,O_L1_LC
  Bus Selector8 : BusSelector  OutputSignals=O_R1_C0,O_R1_C1,O_R1_C2,O_R1_C3,O_R1_VR,O_R1_Q,O_R1_Type,O_R1_W,O_R1_TLC,O_R1_LC
  Cast To Single{1..4,7..8,10..14,17..18,20..24,27..28,30..34,37..38,40..46,49..50,52..57,60..61,63..68,71..72,74..75,78..79} (56 alike) : DataTypeConversion  OutDataTypeStr=single
  Cast To Single{5..6,9,15..16,19,25..26,29,35..36,39,47..48,51,58..59,62,69..70,73,76..77,80} (24 alike) : DataTypeConversion  OutDataTypeStr=uint8
  Constant : Constant  OutDataTypeStr=uint8
  Subsystem : Subsystem
  Subsystem1 : Subsystem
  Subsystem2 : Subsystem
  Subsystem4 : Subsystem
  Switch : Switch  Criteria=u2 > Threshold
  bsL0Info : Outport
  bsR0Info : Outport  Port=2
  bsL1Info : Outport  Port=3
  bsR1Info : Outport  Port=4
  wires:
  Cast To Single71/1 -> Bus Creator2/8  "L0_W"
  Cast To Single73/1 -> Bus Creator5/10  "R1_LC"
  Cast To Single70/1 -> Bus Creator5/7  "R1_Type"
  Cast To Single69/1 -> Bus Creator5/6  "R1_Q"
  Cast To Single41/1 -> Bus Creator5/9  "R1_TLC"
  Cast To Single53/1 -> Bus Creator5/4  "R1_C3"
  Cast To Single52/1 -> Bus Creator5/8  "R1_W"
  Cast To Single50/1 -> Bus Creator5/5  "R1_VR"
  Cast To Single49/1 -> Bus Creator5/3  "R1_C2"
  Cast To Single46/1 -> Bus Creator5/1  "R1_C0"
  Cast To Single45/1 -> Bus Creator5/2  "R1_C1"
  Cast To Single74/1 -> Bus Creator4/8  "L1_W"
  Cast To Single63/1 -> Bus Creator4/9  "L1_TLC"
  Cast To Single62/1 -> Bus Creator4/10  "L1_LC"
  Cast To Single79/1 -> Bus Creator4/4  "L1_C3"
  Cast To Single78/1 -> Bus Creator4/5  "L1_VR"
  Cast To Single42/1 -> Bus Creator4/2  "L1_C1"
  Cast To Single43/1 -> Bus Creator4/1  "L1_C0"
  Cast To Single59/1 -> Bus Creator4/7  "L1_Type"
  Cast To Single58/1 -> Bus Creator4/6  "L1_Q"
  Cast To Single44/1 -> Bus Creator4/3  "L1_C2"
  Cast To Single75/1 -> Bus Creator3/8  "R0_W"
  Cast To Single72/1 -> Bus Creator3/9  "R0_TLC"
  Cast To Single60/1 -> Bus Creator3/4  "R0_C3"
  Cast To Single57/1 -> Bus Creator3/5  "R0_VR"
  Cast To Single51/1 -> Bus Creator3/10  "R0_LC"
  Cast To Single48/1 -> Bus Creator3/7  "R0_Type"
  Cast To Single47/1 -> Subsystem/1(R0_Q_In)  "R0_Q"
  Cast To Single55/1 -> Bus Creator3/1  "R0_C0"
  Cast To Single54/1 -> Bus Creator3/2  "R0_C1"
  Cast To Single56/1 -> Bus Creator3/3  "R0_C2"
  Cast To Single80/1 -> Bus Creator2/10  "L0_LC"
  Cast To Single77/1 -> Bus Creator2/7  "L0_Type"
  Cast To Single68/1 -> Bus Creator2/9  "L0_TLC"
  Cast To Single76/1 -> Subsystem4/1(L0_Q_In)  "L0_Q"
  Cast To Single64/1 -> Bus Creator2/1  "L0_C0"
  Cast To Single65/1 -> Bus Creator2/3  "L0_C2"
  Cast To Single67/1 -> Bus Creator2/4  "L0_C3"
  Cast To Single66/1 -> Bus Creator2/5  "L0_VR"
  Cast To Single61/1 -> Bus Creator2/2  "L0_C1"
  Bus Creator7/1 -> Bus Creator1/2  "bsR0Info"
  Cast To Single34/1 -> Bus Creator8/9  "L0_TLC"
  Bus Creator15/1 -> Bus Creator1/4  "bsR1Info"
  Cast To Single8/1 -> Bus Creator16/4  "L1_C3"
  Cast To Single29/1 -> Bus Creator16/10  "L1_LC"
  Cast To Single3/1 -> Bus Creator16/9  "L1_TLC"
  Cast To Single18/1 -> Bus Creator15/5  "R1_VR"
  Cast To Single39/1 -> Bus Creator15/10  "R1_LC"
  Cast To Single19/1 -> Bus Creator7/10  "R0_LC"
  Cast To Single12/1 -> Bus Creator16/3  "L1_C2"
  Cast To Single4/1 -> Bus Creator16/8  "L1_W"
  Cast To Single38/1 -> Bus Creator7/9  "R0_TLC"
  Cast To Single11/1 -> Bus Creator16/1  "L1_C0"
  Cast To Single15/1 -> Subsystem1/1(R0_Q_In)  "R0_Q"
  Cast To Single7/1 -> Bus Creator16/5  "L1_VR"
  Cast To Single24/1 -> Bus Creator7/5  "R0_VR"
  Cast To Single20/1 -> Bus Creator15/4  "R1_C3"
  Cast To Single26/1 -> Bus Creator16/7  "L1_Type"
  Cast To Single14/1 -> Bus Creator15/1  "R1_C0"
  Cast To Single13/1 -> Bus Creator15/2  "R1_C1"
  Bus Creator16/1 -> Bus Creator1/3  "bsL1Info"
  Cast To Single23/1 -> Bus Creator7/3  "R0_C2"
  Cast To Single21/1 -> Bus Creator7/2  "R0_C1"
  Cast To Single1/1 -> Bus Creator15/9  "R1_TLC"
  Cast To Single28/1 -> Bus Creator8/2  "L0_C1"
  Cast To Single35/1 -> Bus Creator15/6  "R1_Q"
  Cast To Single16/1 -> Bus Creator7/7  "R0_Type"
  Cast To Single6/1 -> Bus Creator8/7  "L0_Type"
  Cast To Single5/1 -> Subsystem2/1(L0_Q_In)  "L0_Q"
  Cast To Single33/1 -> Bus Creator8/4  "L0_C3"
  Cast To Single30/1 -> Bus Creator8/1  "L0_C0"
  Cast To Single31/1 -> Bus Creator8/3  "L0_C2"
  Cast To Single9/1 -> Bus Creator8/10  "L0_LC"
  Cast To Single36/1 -> Bus Creator15/7  "R1_Type"
  Cast To Single17/1 -> Bus Creator15/3  "R1_C2"
  Cast To Single25/1 -> Bus Creator16/6  "L1_Q"
  Cast To Single22/1 -> Bus Creator7/1  "R0_C0"
  Bus Creator8/1 -> Bus Creator1/1  "bsL0Info"
  Cast To Single40/1 -> Bus Creator7/8  "R0_W"
  Cast To Single37/1 -> Bus Creator8/8  "L0_W"
  Cast To Single32/1 -> Bus Creator8/5  "L0_VR"
  Cast To Single10/1 -> Bus Creator16/2  "L1_C1"
  Cast To Single27/1 -> Bus Creator7/4  "R0_C3"
  Cast To Single2/1 -> Bus Creator15/8  "R1_W"
  bsOriL0Info/1 -> Bus Selector1/1
  Bus Selector1/1 -> Cast To Single30/1  "<O_L0_C0>"
  Bus Selector1/2 -> Cast To Single28/1  "<O_L0_C1>"
  Bus Selector1/3 -> Cast To Single31/1  "<O_L0_C2>"
  Bus Selector1/4 -> Cast To Single33/1  "<O_L0_C3>"
  Bus Selector1/5 -> Cast To Single32/1  "<O_L0_VR>"
  Bus Selector1/6 -> Cast To Single5/1  "<O_L0_Q>"
  Bus Selector1/7 -> Cast To Single6/1  "<O_L0_Type>"
  Bus Selector1/8 -> Cast To Single37/1  "<O_L0_W>"
  Bus Selector1/9 -> Cast To Single34/1  "<O_L0_TLC>"
  Bus Selector1/10 -> Cast To Single9/1  "<O_L0_LC>"
  bsOriR0Info/1 -> Bus Selector6/1
  Bus Selector6/1 -> Cast To Single22/1  "<O_R0_C0>"
  Bus Selector6/2 -> Cast To Single21/1  "<O_R0_C1>"
  Bus Selector6/3 -> Cast To Single23/1  "<O_R0_C2>"
  Bus Selector6/4 -> Cast To Single27/1  "<O_R0_C3>"
  Bus Selector6/5 -> Cast To Single24/1  "<O_R0_VR>"
  Bus Selector6/6 -> Cast To Single15/1  "<O_R0_Q>"
  Bus Selector6/7 -> Cast To Single16/1  "<O_R0_Type>"
  Bus Selector6/8 -> Cast To Single40/1  "<O_R0_W>"
  Bus Selector6/9 -> Cast To Single38/1  "<O_R0_TLC>"
  Bus Selector6/10 -> Cast To Single19/1  "<O_R0_LC>"
  bsOriL1Info/1 -> Bus Selector7/1
  Bus Selector7/1 -> Cast To Single11/1  "<O_L1_C0>"
  Bus Selector7/2 -> Cast To Single10/1  "<O_L1_C1>"
  Bus Selector7/3 -> Cast To Single12/1  "<O_L1_C2>"
  Bus Selector7/4 -> Cast To Single8/1  "<O_L1_C3>"
  Bus Selector7/5 -> Cast To Single7/1  "<O_L1_VR>"
  Bus Selector7/6 -> Cast To Single25/1  "<O_L1_Q>"
  Bus Selector7/7 -> Cast To Single26/1  "<O_L1_Type>"
  Bus Selector7/8 -> Cast To Single4/1  "<O_L1_W>"
  Bus Selector7/9 -> Cast To Single3/1  "<O_L1_TLC>"
  Bus Selector7/10 -> Cast To Single29/1  "<O_L1_LC>"
  bsOriR1Info/1 -> Bus Selector8/1
  Bus Selector8/1 -> Cast To Single14/1  "<O_R1_C0>"
  Bus Selector8/2 -> Cast To Single13/1  "<O_R1_C1>"
  Bus Selector8/3 -> Cast To Single17/1  "<O_R1_C2>"
  Bus Selector8/4 -> Cast To Single20/1  "<O_R1_C3>"
  Bus Selector8/5 -> Cast To Single18/1  "<O_R1_VR>"
  Bus Selector8/6 -> Cast To Single35/1  "<O_R1_Q>"
  Bus Selector8/7 -> Cast To Single36/1  "<O_R1_Type>"
  Bus Selector8/8 -> Cast To Single2/1  "<O_R1_W>"
  Bus Selector8/9 -> Cast To Single1/1  "<O_R1_TLC>"
  Bus Selector8/10 -> Cast To Single39/1  "<O_R1_LC>"
  Bus Creator2/1 -> Bus Creator/1  "bsL0Info"
  Bus Creator3/1 -> Bus Creator/2  "bsR0Info"
  Bus Creator4/1 -> Bus Creator/3  "bsL1Info"
  Bus Creator/1 -> Switch/1
  Bus Creator1/1 -> Switch/3
  Constant/1 -> Switch/2
  Switch/1 -> Bus Selector/1
  Bus Selector4/5 -> Cast To Single78/1  "<L1_VR>"
  Bus Selector4/2 -> Cast To Single42/1  "<L1_C1>"
  Bus Selector3/5 -> Cast To Single57/1  "<R0_VR>"
  Subsystem4/1(L0_Q) -> Bus Creator2/6
  Bus Selector4/1 -> Cast To Single43/1  "<L1_C0>"
  Bus Selector2/4 -> Cast To Single67/1  "<L0_C3>"
  Bus Selector2/6 -> Cast To Single76/1  "<L0_Q>"
  bsFusR1Info/1 -> Bus Selector5/1
  bsFusL1Info/1 -> Bus Selector4/1
  bsFusR0Info/1 -> Bus Selector3/1
  Bus Selector4/7 -> Cast To Single59/1  "<L1_Type>"
  bsFusL0Info/1 -> Bus Selector2/1
  Bus Selector3/10 -> Cast To Single51/1  "<R0_LC>"
  Bus Selector5/10 -> Cast To Single73/1  "<R1_LC>"
  Bus Selector2/3 -> Cast To Single65/1  "<L0_C2>"
  Bus Selector5/1 -> Cast To Single46/1  "<R1_C0>"
  Bus Selector3/8 -> Cast To Single75/1  "<R0_W>"
  Bus Selector3/7 -> Cast To Single48/1  "<R0_Type>"
  Bus Selector3/9 -> Cast To Single72/1  "<R0_TLC>"
  Bus Selector3/3 -> Cast To Single56/1  "<R0_C2>"
  Bus Selector2/10 -> Cast To Single80/1  "<L0_LC>"
  Bus Selector5/7 -> Cast To Single70/1  "<R1_Type>"
  Bus Selector2/9 -> Cast To Single68/1  "<L0_TLC>"
  Bus Selector5/6 -> Cast To Single69/1  "<R1_Q>"
  Bus Selector5/5 -> Cast To Single50/1  "<R1_VR>"
  Bus Selector2/5 -> Cast To Single66/1  "<L0_VR>"
  Bus Selector2/1 -> Cast To Single64/1  "<L0_C0>"
  Bus Selector4/10 -> Cast To Single62/1  "<L1_LC>"
  Bus Selector3/4 -> Cast To Single60/1  "<R0_C3>"
  Bus Selector2/8 -> Cast To Single71/1  "<L0_W>"
  Bus Selector3/2 -> Cast To Single54/1  "<R0_C1>"
  Bus Selector3/1 -> Cast To Single55/1  "<R0_C0>"
  Bus Selector2/2 -> Cast To Single61/1  "<L0_C1>"
  Bus Selector4/4 -> Cast To Single79/1  "<L1_C3>"
  Bus Selector4/6 -> Cast To Single58/1  "<L1_Q>"
  Bus Selector4/9 -> Cast To Single63/1  "<L1_TLC>"
  Bus Selector2/7 -> Cast To Single77/1  "<L0_Type>"
  Subsystem/1(R0_Q) -> Bus Creator3/6
  Bus Selector3/6 -> Cast To Single47/1  "<R0_Q>"
  Bus Selector5/9 -> Cast To Single41/1  "<R1_TLC>"
  Bus Selector5/4 -> Cast To Single53/1  "<R1_C3>"
  Bus Creator5/1 -> Bus Creator/4  "bsR1Info"
  Bus Selector5/8 -> Cast To Single52/1  "<R1_W>"
  Bus Selector5/2 -> Cast To Single45/1  "<R1_C1>"
  Bus Selector5/3 -> Cast To Single49/1  "<R1_C2>"
  Bus Selector4/8 -> Cast To Single74/1  "<L1_W>"
  Bus Selector4/3 -> Cast To Single44/1  "<L1_C2>"
  Bus Selector/1 -> bsL0Info/1  "<bsL0Info>"
  Bus Selector/2 -> bsR0Info/1  "<bsR0Info>"
  Bus Selector/3 -> bsL1Info/1  "<bsL1Info>"
  Bus Selector/4 -> bsR1Info/1  "<bsR1Info>"
  Subsystem2/1(L0_Q) -> Bus Creator8/6
  Subsystem1/1(R0_Q) -> Bus Creator7/6

== system D53_LKAS_JLU_20200909_1612/LL/LL Inputs Mapping/bsLaneInfo/LanesReconstruct  ==
  bsL0Info : Inport
  bsR0Info : Inport  Port=2
  bsL1Info : Inport  Port=3
  bsR1Info : Inport  Port=4
  Bus Selector5 : BusSelector  OutputSignals=L0_Q
  Bus Selector6 : BusSelector  OutputSignals=R0_Q
  LaneReconstructSM : Stateflow chart  TreatAsAtomicUnit=on
  Left 1Lane Reconstruct (Lft1LaneR) : Subsystem
  Left Lane Reconstruct (LftLaneR) : Subsystem
  Right 1Lane Reconstruct (Rgt1LaneR) : Subsystem
  Right Lane Reconstruct (RgtLaneR) : Subsystem
  RoadSide Offset : Subsystem
  Switch : Switch  Criteria=u2 > Threshold
  Switch1 : Switch  Criteria=u2 > Threshold
  bsL0InfoR : Outport
  bsR0InfoR : Outport  Port=2
  bsL1InfoR : Outport  Port=3
  bsR1InfoR : Outport  Port=4
  wires:
  RoadSide Offset/2(bsR0Infoout) -> Bus Selector6/1, Left Lane Reconstruct (LftLaneR)/2(bsR0Info), Right Lane Reconstruct (RgtLaneR)/2(bsR0Info), Switch/1
  RoadSide Offset/1(bsL0Infoout) -> Bus Selector5/1, Right Lane Reconstruct (RgtLaneR)/1(bsL0Info), Switch1/1, Left Lane Reconstruct (LftLaneR)/3(bsL0Info)
  bsL0Info/1 -> RoadSide Offset/1(bsL0Info)
  bsR0Info/1 -> RoadSide Offset/2(bsR0Info)
  [LftFlg] -> Switch1/2
  [RgtFlg] -> Switch/2
  [LftFlg] -> Left 1Lane Reconstruct (Lft1LaneR)/1(stFlag)
  [RgtFlg] -> Right 1Lane Reconstruct (Rgt1LaneR)/1(stFlag)
  Left 1Lane Reconstruct (Lft1LaneR)/1(bsL1InfoR) -> bsL1InfoR/1
  Right 1Lane Reconstruct (Rgt1LaneR)/1(bsL1InfoR) -> bsR1InfoR/1
  bsR1Info/1 -> Right 1Lane Reconstruct (Rgt1LaneR)/2(bsR1Info)
  LaneReconstructSM/3(LaneRSM_stRgtFlg) -> [RgtFlg]
  LaneReconstructSM/2(LaneRSM_stLftFlg) -> [LftFlg]
  LaneReconstructSM/1(LaneRSM_stRoadFlg) -> [RoadFlg]
  Switch1/1 -> bsL0InfoR/1
  Switch/1 -> bsR0InfoR/1
  Right Lane Reconstruct (RgtLaneR)/1(bsR0InfoR) -> Switch/3
  Left Lane Reconstruct (LftLaneR)/1(bsL0InfoR) -> Switch1/3
  RoadSide Offset/3(lRoadW) -> Right Lane Reconstruct (RgtLaneR)/3(lRoadW), Left Lane Reconstruct (LftLaneR)/1(lRoadW), [RoadWidth]
  Bus Selector5/1 -> LaneReconstructSM/1(LaneRSM_stL0Ql)  "<L0_Q>"
  Bus Selector6/1 -> LaneReconstructSM/2(LaneRSM_stR0Ql)  "<R0_Q>"
  bsL1Info/1 -> Left 1Lane Reconstruct (Lft1LaneR)/2(bsL1Info)

== system D53_LKAS_JLU_20200909_1612/LL/LLOn/LDW/Heading Angle Detection (HdAgDet) ==
  HdAgDet_stLDWActvFlg : Inport
  HdAgDet_phiHdAgLft : Inport  Port=2
  HdAgDet_phiHdAgRgt : Inport  Port=3
  HdAgDet_phiHdAgThres_C : Inport  Port=4
  Constant : Constant  Value=5  OutDataTypeStr=single
  If : If  IfExpression=u1==1  ElseIfExpressions=u1==2
  If Action Subsystem : Subsystem  TreatAsAtomicUnit=on
  If Action Subsystem1 : Subsystem  TreatAsAtomicUnit=on
  If Action Subsystem2 : Subsystem  TreatAsAtomicUnit=on
  Merge : Merge  Inputs=3  InitialOutput=0
  Relational Operator : RelationalOperator  OutDataTypeStr=boolean  RndMeth=Nearest
  Sum Condition : Subsystem
  HdAgDet_stHdAgDetFlg : Outport
  wires:
  Constant/1 -> Sum Condition/2(Sum)
  Relational Operator/1 -> Sum Condition/Enable, Sum Condition/1(In)
  Sum Condition/1(Out) -> HdAgDet_stHdAgDetFlg/1
  HdAgDet_phiHdAgThres_C/1 -> Relational Operator/2
  Merge/1 -> Relational Operator/1
  HdAgDet_stLDWActvFlg/1 -> If/1
  HdAgDet_phiHdAgRgt/1 -> If Action Subsystem1/1(In1)
  HdAgDet_phiHdAgLft/1 -> If Action Subsystem/1(In1)
  If/3 -> If Action Subsystem2/Action
  If Action Subsystem2/1(Out1) -> Merge/3
  If/2 -> If Action Subsystem1/Action
  If Action Subsystem1/1(Out1) -> Merge/2
  If Action Subsystem/1(Out1) -> Merge/1
  If/1 -> If Action Subsystem/Action

== system D53_LKAS_JLU_20200909_1612/LL/LLOn/LKA/Driver Torque Addition (DTA) ==
  DTA_bsInInfoSyn : Inport
  DTA_bsLFClb : Inport  Port=2
  Bus Selector : BusSelector  OutputSignals=LL_LKASWAClb.LL_LKASWASyn_TrqSwaAddSwt
  Compare To Constant : simulink/Logic and Bit Operations/Compare To Constant  relop=>  const=0  OutDataTypeStr=boolean
  Subsystem : Subsystem
  Subsystem1 : Subsystem
  DTA_phiDTASWACmd : Outport
  DTA_M : Outport  Port=2
  wires:
  Compare To Constant/1 -> Subsystem/Enable
  Bus Selector/1 -> Compare To Constant/1  "<LL_LKASWASyn_TrqSwaAddSwt>"
  Subsystem1/1(Out1) -> DTA_M/1
  Subsystem/1(Out1) -> DTA_phiDTASWACmd/1
  DTA_bsLFClb/1 -> Bus Selector/1, Subsystem/2(DTA_bsLFClb), Subsystem1/2(DTA_bsLFClb)
  DTA_bsInInfoSyn/1 -> Subsystem1/1(DTA_bsInInfoSyn), Subsystem/1(DTA_bsInInfoSyn)
  [LKA_SampleTime] -> Subsystem/3(LKA_SampleTime)

== system D53_LKAS_JLU_20200909_1612/LL/LLOn/LKA/LKA Exit Processing (LKAExPrcs) ==
  LKAExPrcs_bsInInfoSyn : Inport
  LKAExPrcs_bsLKAInPInfo : Inport  Port=2
  LKAExPrcs_bsLKAClb : Inport  Port=3
  LKAExPrcs_PlanT1 : Inport  Port=4
  Cast To Single : DataTypeConversion  OutDataTypeStr=single
  Exit Time 1 : Subsystem
  Exit Time 2 : Subsystem
  Exit Time 3 : Subsystem
  Fcn : Fcn  Expr=u(3)*(u(3)==1)*3+u(2)*(u(3)==0)*2+u(1)*(u(2)==0&&u(3)==0)
  Logical Operator3 : Logic  Operator=OR  Inputs=3  AllPortsSameDT=off  OutDataTypeStr=boolean
  Mux : Mux  Inputs=3
  LKAExPrcs_stExFlg : Outport
  LKAExPrcs_stExNum : Outport  Port=2
  wires:
  Cast To Single/1 -> Fcn/1
  Fcn/1 -> LKAExPrcs_stExNum/1  "ExNum"
  Mux/1 -> Cast To Single/1
  LKAExPrcs_PlanT1/1 -> Exit Time 3/4(T1), Exit Time 2/4(T1)
  LKAExPrcs_bsLKAClb/1 -> Exit Time 3/3(bsLKAClb), Exit Time 2/2(bsLKAClb), Exit Time 1/2(bsLKAClb)
  LKAExPrcs_bsLKAInPInfo/1 -> Exit Time 1/1(bsLKAInPInfo), Exit Time 2/3(bsLKAInPInfo), Exit Time 3/2(bsLKAInPInfo)
  Exit Time 3/1(Exit3) -> Logical Operator3/3, Mux/3
  Exit Time 2/1(Exit2) -> Logical Operator3/2, Mux/2
  Exit Time 1/1(Exit1) -> Logical Operator3/1, Mux/1
  Logical Operator3/1 -> LKAExPrcs_stExFlg/1
  LKAExPrcs_bsInInfoSyn/1 -> Exit Time 2/1(bsInInfoSyn), Exit Time 3/1(bsInInfoSyn)

== system D53_LKAS_JLU_20200909_1612/LL/LLOn/LKA/LKA Motion Planning (LKAMP)  ==
  LKAMP_bsInInfoSyn : Inport
  LKAMP_stLKAActvFlg : Inport  Port=2
  LKAMP_bsLKAInPInfo : Inport  Port=3
  LKAMP_bsLKAClb : Inport  Port=4
  LLClb_bsConstantClb : Inport  Port=5
  Add : Sum  OutDataTypeStr=uint8
  Bus Selector : BusSelector  OutputSignals=MPInP_vVehSpdIni
  Bus Selector1 : BusSelector  OutputSignals=bsVehMovInfo.ESC_VehSpd
  Bus Selector2 : BusSelector  OutputSignals=LKA_CarWidth
  Bus Selector3 : BusSelector  OutputSignals=LL_HdAgExT_C,LL_LSpdCompT_C
  Bus Selector4 : BusSelector  OutputSignals=bsVehMovInfo.ESC_VehSpd
  Bus Selector5 : BusSelector  OutputSignals=LW_LaneWidth
  Constant : Constant  OutDataTypeStr=uint8  SampleTime=-1
  Constant19 : Constant  OutDataTypeStr=uint8  SampleTime=-1
  If : If  NumInputs=2  IfExpression=u1==u2  ShowElse=off
  LKA Motion Planning Calculation (LKAMPCal) : Subsystem  Description=|
      | Block Name: LKA Motion Planning Calculation
      | Ab.: LKAMPCal
      | No.: 1.2.3.2
      | Rev: 0.0.1
      | Update Date: 19-3-26
      settings: RTWSystemCode=Nonreusable function
  Memory1 : Memory  InheritSampleTime=on
  Motion Planning Input Processing (MPInP) : Subsystem  Description=|
      | Block Name: Motion Planning Input Processing
      | Ab.: MPInP
      | No.: 1.2.3.1
      | Rev: 0.0.1
      | Update Date: 19-3-26
  Nominal Time Calculation (NomTCalc) : Subsystem  Description=|
      | Block Name: Nominal Time Calculation
      | Ab.: NomTCalc
      | No.: 1.2.3.3
      | Rev: 0.0.1
      | Update Date: 19-3-26
  Saturation1 : Saturate  UpperLimit=5  LowerLimit=0  OutDataTypeStr=uint8
  Saturation6 : Saturate  UpperLimit=2  LowerLimit=0.2
  Steering Wheel Angle Command Calculation (SWACmdCal) : Subsystem  Description=|
      | Block Name: Steering Wheel Angle Command Calculation
      | Ab.: SWACmdCal
      | No.: 1.2.3.4
      | Rev: 0.0.1
      | Update Date: 19-3-26
  Switching Condition (SwtCon) : Subsystem
  LKAMP_phiSWACmd : Outport
  LKAMP_tiT1 : Outport  Port=2
  LKAMP_tiT2 : Outport  Port=3
  wires:
  Bus Selector5/1 -> Switching Condition (SwtCon)/4(SwtCon_lLaneWidth_C)  "<LW_LaneWidth>"
  Saturation6/1 -> LKAMP_tiT1/1
  LKAMP_bsInInfoSyn/1 -> Bus Selector4/1, Bus Selector1/1, Motion Planning Input Processing (MPInP)/4(MPInP_bsInInfoSyn)
  Bus Selector3/2 -> Switching Condition (SwtCon)/7(SwtCon_tiLSpdCompT_C)  "<LL_LSpdCompT_C>"
  LLClb_bsConstantClb/1 -> Bus Selector2/1, LKA Motion Planning Calculation (LKAMPCal)/3(LLClb_bsConstantClb)
  LKAMP_bsLKAInPInfo/1 -> Motion Planning Input Processing (MPInP)/3(MPInP_bsLKAInPInfo), Switching Condition (SwtCon)/2(SwtCon_bsLKAInPInfo), Bus Selector5/1
  Bus Selector2/1 -> Switching Condition (SwtCon)/5(SwtCon_lCarWidth_C)  "<LKA_CarWidth>"
  LKAMP_bsLKAClb/1 -> LKA Motion Planning Calculation (LKAMPCal)/2(LKAMPCal_bsLKAClb), Bus Selector3/1
  LKAMP_stLKAActvFlg/1 -> Motion Planning Input Processing (MPInP)/1(MPInP_stLKAActvFlg), Switching Condition (SwtCon)/1(SwtCon_stLKAActvFlg)
  Bus Selector4/1 -> Switching Condition (SwtCon)/3(SwtCon_vVehSpd)  "<ESC_VehSpd>"
  Bus Selector3/1 -> Switching Condition (SwtCon)/6(SwtCon_tiHdAgExTime_C)  "<LL_HdAgExT_C>"
  Saturation1/1 -> If/1, Memory1/1
  Add/1 -> Saturation1/1
  Constant19/1 -> If/2
  Constant/1 -> Add/1
  Memory1/1 -> Add/2
  If/1 -> LKA Motion Planning Calculation (LKAMPCal)/Action
  LKA Motion Planning Calculation (LKAMPCal)/1(LKAMPCal_bsLKAMPCalOut) -> Steering Wheel Angle Command Calculation (SWACmdCal)/1(SWACmdCal_bsK1K2DetOut)
  Switching Condition (SwtCon)/1(SwtCon_phiHdAgMax) -> Motion Planning Input Processing (MPInP)/2(MPInP_phiHdAgMax)
  Nominal Time Calculation (NomTCalc)/1(NomTCalc_tiNomT) -> Steering Wheel Angle Command Calculation (SWACmdCal)/3(SWACmdCal_tiNomT)
  Bus Selector1/1 -> Nominal Time Calculation (NomTCalc)/1(NomTCalc_vVehSpd)  "<ESC_VehSpd>"
  Bus Selector/1 -> Nominal Time Calculation (NomTCalc)/2(NomTCalc_vVehSpdIni)  "<MPInP_vVehSpdIni>"
  Steering Wheel Angle Command Calculation (SWACmdCal)/1(SWACmdCal_phiSWACmd) -> LKAMP_phiSWACmd/1
  Steering Wheel Angle Command Calculation (SWACmdCal)/2(SWACmdCal_tiT1) -> Saturation6/1
  Motion Planning Input Processing (MPInP)/1(MPInP_bsMPInPInfo) -> LKA Motion Planning Calculation (LKAMPCal)/1(LKAMPCal_bsLKAInPInfo), Bus Selector/1, Steering Wheel Angle Command Calculation (SWACmdCal)/2(SWACmdCal_bsLKAInPInfo)  "LKAMP_bsMPInPInfo"
  Steering Wheel Angle Command Calculation (SWACmdCal)/3(SWACmdCal_tiT2) -> LKAMP_tiT2/1
